simulink model "part_2"  (R2025b)
settings: Solver=VariableStepAuto  StartTime=0.0  StopTime=10.0  RelTol=1e-3
libraries: dspxfrm3 x1
settings Model: Creator=Ultor  LastModifiedBy=Ultor

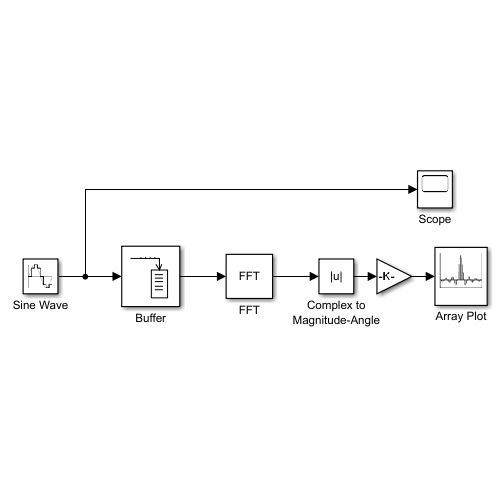
[thumbnail: Simulink's stored preview of the top-level diagram]
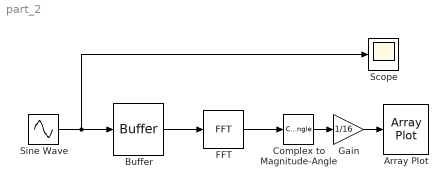
== system part_2 ==
  Array Plot : ArrayPlot  WindowPosition=[657.000000,116.000000,1019.000000,725.000000,]  Visible=on  ScopeFrameLocation=window  YLimits=[-0.0625 0.5625]
  Buffer : Buffer  N=16  OutputFrames=off
  Complex to Magnitude-Angle : ComplexToMagnitudeAngle  Output=Magnitude
  FFT : dspxfrm3/FFT  FFTImplementation=Auto  CompMethod=Table lookup  TableOpt=NEW  TableOptActive=Speed  BitRevOrder=off  Normalize=off  InheritFFTLength=on  FFTLength=64  WrapInput=on  roundingMode=Ceiling  overflowMode=off  firstCoeffDataTypeStr=Inherit: Same word length as input  firstCoeffLastDataTypeStr=Inherit: Same word length as input  outputMin=[]  outputMax=[]
  Gain : Gain  Gain=1/16
  Scope : Scope
      settings: ActiveDisplayYMinimum=-1.25  ActiveDisplayYMaximum=1.25  DataLoggingVariableName=ScopeData2  DataLoggingSaveFormat=Array
  Sine Wave : Sin  Frequency=2*pi*110  SampleTime=1/440
  wires:
  FFT/1 -> Complex to Magnitude-Angle/1
  Sine Wave/1 -> Buffer/1, Scope/1
  Buffer/1 -> FFT/1
  Complex to Magnitude-Angle/1 -> Gain/1
  Gain/1 -> Array Plot/1
